simulink model "trapezgeschw_mit_statemachine"  (R2023b)
settings: Solver=ode5  StartTime=0.0  StopTime=10.0  FixedStep=1e-3  RelTol=1e-3
undefined symbols (not defined in the file or in its folder): DiscIntNeverNeededParam
settings Model: Creator=pucher  LastModifiedBy=Flo
settings SolverCC: AlgebraicLoopSolver=TrustRegion
settings DebuggingCC: UnconnectedInputMsg=warning  UnconnectedOutputMsg=warning  UnconnectedLineMsg=warning  ArithmeticOperatorsInVariantConditions=warning
settings ModelReferenceCC: EnableRefExpFcnMdlSchedulingChecks=on
settings SFSimCC: CustomCodeUndefinedFunction=UseInterfaceOnly

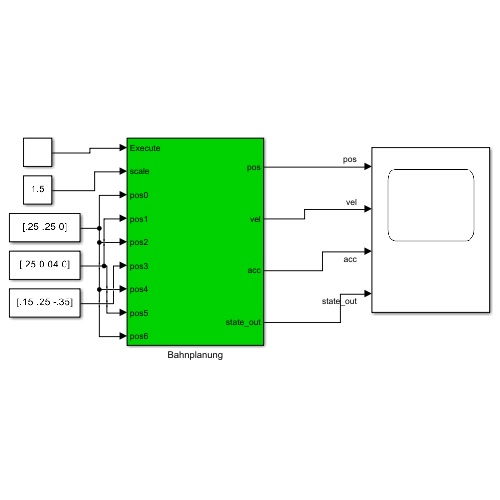
[thumbnail: Simulink's stored preview of the top-level diagram]
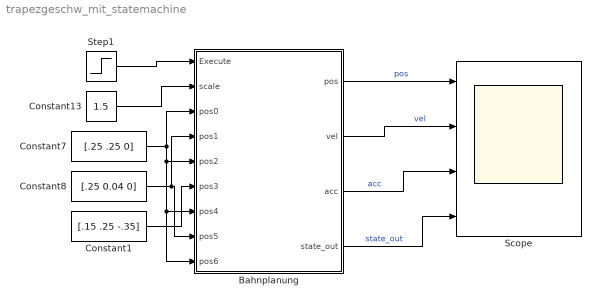
== system trapezgeschw_mit_statemachine ==
  Bahnplanung : Subsystem
  Constant1 : Constant  Value=[.15 .25 -.35]
  Constant13 : Constant  Value=1.5
  Constant7 : Constant  Value=[.25 .25 0]
  Constant8 : Constant  Value=[.25 0.04 0]
  Scope : Scope  NumInputPorts=4
  Step1 : Step
  wires:
  Constant7/1 -> Bahnplanung/9(pos6), Bahnplanung/7(pos4), Bahnplanung/5(pos2), Bahnplanung/3(pos0)
  Step1/1 -> Bahnplanung/1(Execute)
  Constant8/1 -> Bahnplanung/8(pos5), Bahnplanung/4(pos1)
  Bahnplanung/1(pos) -> Scope/1  "pos"
  Bahnplanung/2(vel) -> Scope/2  "vel"
  Bahnplanung/3(acc) -> Scope/3  "acc"
  Bahnplanung/4(state_out) -> Scope/4  "state_out"
  Constant13/1 -> Bahnplanung/2(scale)
  Constant1/1 -> Bahnplanung/6(pos3)

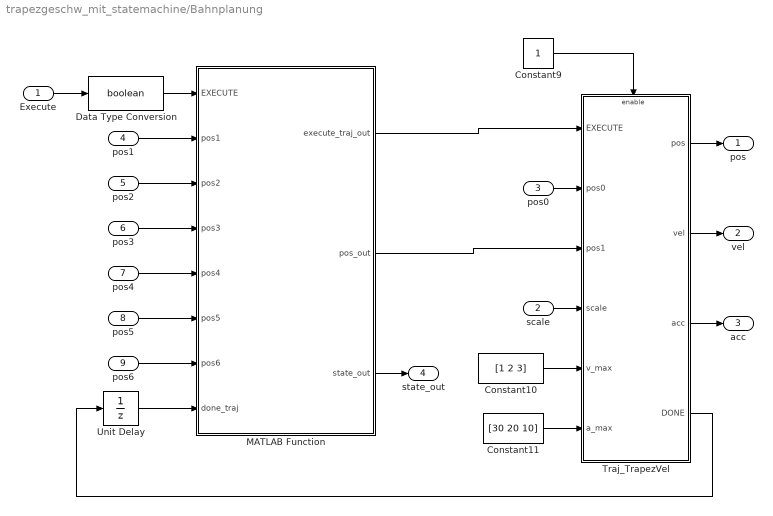
== system trapezgeschw_mit_statemachine/Bahnplanung ==
  Execute : Inport
  scale : Inport  Port=2
  pos0 : Inport  Port=3
  pos1 : Inport  Port=4
  pos2 : Inport  Port=5
  pos3 : Inport  Port=6
  pos4 : Inport  Port=7
  pos5 : Inport  Port=8
  pos6 : Inport  Port=9
  Constant10 : Constant  Value=[1 2 3]
  Constant11 : Constant  Value=[30 20 10]
  Constant9 : Constant
  Data Type Conversion : DataTypeConversion  OutDataTypeStr=boolean  SaturateOnIntegerOverflow=off  RndMeth=Floor
  MATLAB Function : MATLAB Function  TreatAsAtomicUnit=on
  Traj_TrapezVel : Subsystem
  Unit Delay : UnitDelay  SampleTime=-1  HasFrameUpgradeWarning=on
  pos : Outport
  vel : Outport  Port=2
  acc : Outport  Port=3
  state_out : Outport  Port=4
  wires:
  MATLAB Function/1(execute_traj_out) -> Traj_TrapezVel/1(EXECUTE)
  Constant10/1 -> Traj_TrapezVel/5(v_max)
  Unit Delay/1 -> MATLAB Function/8(done_traj)
  Constant9/1 -> Traj_TrapezVel/Enable
  scale/1 -> Traj_TrapezVel/4(scale)
  Traj_TrapezVel/4(DONE) -> Unit Delay/1
  Data Type Conversion/1 -> MATLAB Function/1(EXECUTE)
  Constant11/1 -> Traj_TrapezVel/6(a_max)
  Traj_TrapezVel/1(pos) -> pos/1
  Traj_TrapezVel/2(vel) -> vel/1
  MATLAB Function/2(pos_out) -> Traj_TrapezVel/3(pos1)
  MATLAB Function/3(state_out) -> state_out/1
  pos2/1 -> MATLAB Function/3(pos2)
  Execute/1 -> Data Type Conversion/1
  Traj_TrapezVel/3(acc) -> acc/1
  pos1/1 -> MATLAB Function/2(pos1)
  pos0/1 -> Traj_TrapezVel/2(pos0)
  pos4/1 -> MATLAB Function/5(pos4)
  pos5/1 -> MATLAB Function/6(pos5)
  pos3/1 -> MATLAB Function/4(pos3)
  pos6/1 -> MATLAB Function/7(pos6)

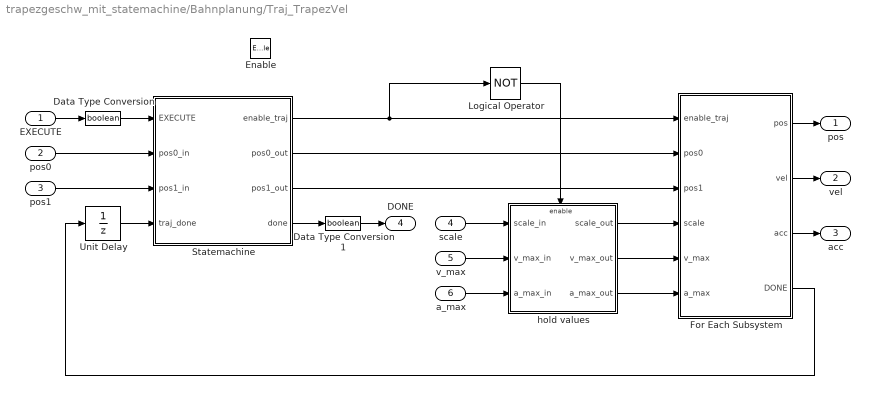
== system trapezgeschw_mit_statemachine/Bahnplanung/Traj_TrapezVel ==
  EXECUTE : Inport
  pos0 : Inport  Port=2
  pos1 : Inport  Port=3
  scale : Inport  Port=4
  v_max : Inport  Port=5
  a_max : Inport  Port=6
  Enable : EnablePort  StatesWhenEnabling=reset
  Data Type Conversion : DataTypeConversion  OutDataTypeStr=boolean  SaturateOnIntegerOverflow=off  RndMeth=Floor
  Data Type Conversion1 : DataTypeConversion  OutDataTypeStr=boolean  SaturateOnIntegerOverflow=off  RndMeth=Floor
  For Each Subsystem : Subsystem  TreatAsAtomicUnit=on
  Logical Operator : Logic  Operator=NOT  AllPortsSameDT=off  OutDataTypeStr=boolean
  Statemachine : MATLAB Function  TreatAsAtomicUnit=on
  Unit Delay : UnitDelay  SampleTime=-1  HasFrameUpgradeWarning=on
  hold values : Subsystem  TreatAsAtomicUnit=on
  pos : Outport
  vel : Outport  Port=2
  acc : Outport  Port=3
  DONE : Outport  Port=4  PortDimensions=1
  wires:
  For Each Subsystem/1(pos) -> pos/1
  For Each Subsystem/2(vel) -> vel/1
  For Each Subsystem/3(acc) -> acc/1
  Statemachine/3(pos1_out) -> For Each Subsystem/3(pos1)
  Unit Delay/1 -> Statemachine/4(traj_done)
  EXECUTE/1 -> Data Type Conversion/1
  pos0/1 -> Statemachine/2(pos0_in)
  For Each Subsystem/4(DONE) -> Unit Delay/1
  pos1/1 -> Statemachine/3(pos1_in)
  Data Type Conversion/1 -> Statemachine/1(EXECUTE)
  Statemachine/2(pos0_out) -> For Each Subsystem/2(pos0)
  Statemachine/4(done) -> Data Type Conversion1/1
  Data Type Conversion1/1 -> DONE/1
  scale/1 -> hold values/1(scale_in)
  hold values/1(scale_out) -> For Each Subsystem/4(scale)
  v_max/1 -> hold values/2(v_max_in)
  hold values/2(v_max_out) -> For Each Subsystem/5(v_max)
  a_max/1 -> hold values/3(a_max_in)
  hold values/3(a_max_out) -> For Each Subsystem/6(a_max)
  Logical Operator/1 -> hold values/Enable
  Statemachine/1(enable_traj) -> Logical Operator/1, For Each Subsystem/1(enable_traj)

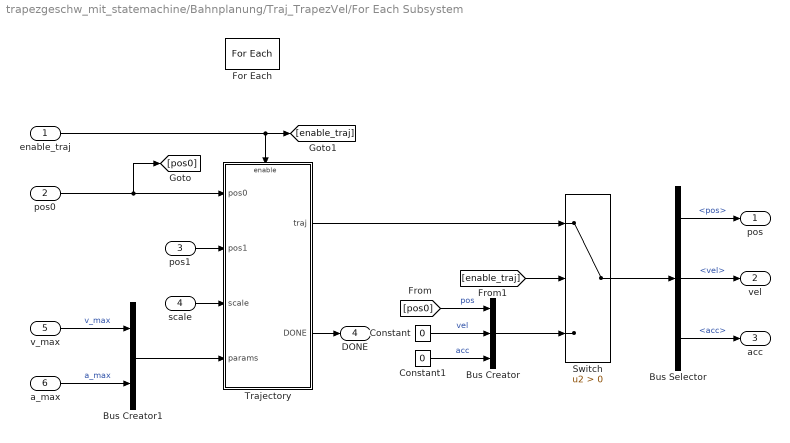
== system trapezgeschw_mit_statemachine/Bahnplanung/Traj_TrapezVel/For Each Subsystem ==
  enable_traj : Inport
  pos0 : Inport  Port=2  Partition=on  PartitionDimension=1  PartitionWidth=1  PartitionOffset=0
  pos1 : Inport  Port=3  Partition=on  PartitionDimension=1  PartitionWidth=1  PartitionOffset=0
  scale : Inport  Port=4
  v_max : Inport  Port=5  Partition=on  PartitionDimension=1  PartitionWidth=1  PartitionOffset=0
  a_max : Inport  Port=6  Partition=on  PartitionDimension=1  PartitionWidth=1  PartitionOffset=0
  Bus Creator : BusCreator  Inputs=3
  Bus Creator1 : BusCreator  Inputs=2
  Bus Selector : BusSelector  OutputSignals=pos,vel,acc
  Constant : Constant  Value=0
  Constant1 : Constant  Value=0
  For Each : ForEach  DisableCoverage=on
  Switch : Switch  Criteria=u2 > Threshold  SaturateOnIntegerOverflow=off  InputSameDT=off
  Trajectory : Subsystem
  pos : Outport  ConcatenationDimension=1
  vel : Outport  Port=2  ConcatenationDimension=1
  acc : Outport  Port=3  ConcatenationDimension=1
  DONE : Outport  Port=4  ConcatenationDimension=1  VectorParamsAs1DForOutWhenUnconnected=off
  wires:
  Constant1/1 -> Bus Creator/3  "acc"
  Constant/1 -> Bus Creator/2  "vel"
  pos1/1 -> Trajectory/2(pos1)
  Bus Creator1/1 -> Trajectory/4(params)
  Trajectory/2(DONE) -> DONE/1
  [enable_traj] -> Switch/2
  Switch/1 -> Bus Selector/1
  Bus Creator/1 -> Switch/3
  pos0/1 -> Trajectory/1(pos0), [pos0]
  Bus Selector/1 -> pos/1  "<pos>"
  v_max/1 -> Bus Creator1/1  "v_max"
  Trajectory/1(traj) -> Switch/1
  scale/1 -> Trajectory/3(scale)
  enable_traj/1 -> [enable_traj], Trajectory/Enable
  Bus Selector/2 -> vel/1  "<vel>"
  Bus Selector/3 -> acc/1  "<acc>"
  a_max/1 -> Bus Creator1/2  "a_max"
  [pos0] -> Bus Creator/1  "pos"

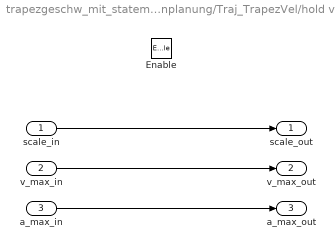
== system trapezgeschw_mit_statemachine/Bahnplanung/Traj_TrapezVel/hold values ==
  scale_in : Inport
  v_max_in : Inport  Port=2
  a_max_in : Inport  Port=3
  Enable : EnablePort
  scale_out : Outport
  v_max_out : Outport  Port=2
  a_max_out : Outport  Port=3
  wires:
  scale_in/1 -> scale_out/1
  v_max_in/1 -> v_max_out/1
  a_max_in/1 -> a_max_out/1

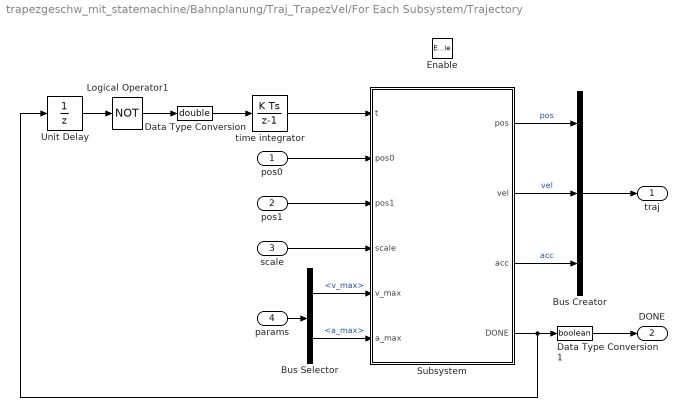
== system trapezgeschw_mit_statemachine/Bahnplanung/Traj_TrapezVel/For Each Subsystem/Trajectory ==
  pos0 : Inport  PortDimensions=1
  pos1 : Inport  Port=2  PortDimensions=1
  scale : Inport  Port=3  PortDimensions=1
  params : Inport  Port=4
  Enable : EnablePort  StatesWhenEnabling=reset
  Bus Creator : BusCreator  Inputs=3
  Bus Selector : BusSelector  OutputSignals=v_max,a_max
  Data Type Conversion : DataTypeConversion  OutDataTypeStr=double  SaturateOnIntegerOverflow=off  RndMeth=Floor
  Data Type Conversion1 : DataTypeConversion  OutDataTypeStr=boolean  SaturateOnIntegerOverflow=off  RndMeth=Floor
  Logical Operator1 : Logic  Operator=NOT  AllPortsSameDT=off  OutDataTypeStr=boolean
  Subsystem : Subsystem
  Unit Delay : UnitDelay  SampleTime=-1  HasFrameUpgradeWarning=on
  time integrator : DiscreteIntegrator  SampleTime=-1  ICPrevOutput=DiscIntNeverNeededParam  ICPrevScaledInput=DiscIntNeverNeededParam
  traj : Outport  VectorParamsAs1DForOutWhenUnconnected=off
  DONE : Outport  Port=2  PortDimensions=1  VectorParamsAs1DForOutWhenUnconnected=off
  wires:
  Data Type Conversion1/1 -> DONE/1
  params/1 -> Bus Selector/1
  Bus Creator/1 -> traj/1
  Logical Operator1/1 -> Data Type Conversion/1
  Unit Delay/1 -> Logical Operator1/1
  Data Type Conversion/1 -> time integrator/1
  Subsystem/4(DONE) -> Unit Delay/1, Data Type Conversion1/1
  time integrator/1 -> Subsystem/1(t)
  pos0/1 -> Subsystem/2(pos0)
  pos1/1 -> Subsystem/3(pos1)
  scale/1 -> Subsystem/4(scale)
  Bus Selector/1 -> Subsystem/5(v_max)  "<v_max>"
  Bus Selector/2 -> Subsystem/6(a_max)  "<a_max>"
  Subsystem/1(pos) -> Bus Creator/1  "pos"
  Subsystem/2(vel) -> Bus Creator/2  "vel"
  Subsystem/3(acc) -> Bus Creator/3  "acc"

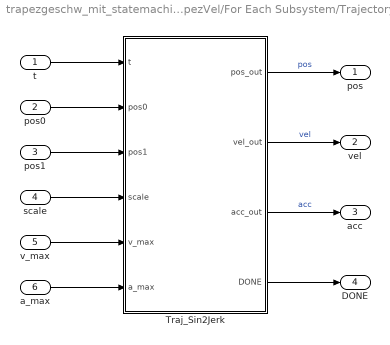
== system trapezgeschw_mit_statemachine/Bahnplanung/Traj_TrapezVel/For Each Subsystem/Trajectory/Subsystem ==
  t : Inport
  pos0 : Inport  Port=2
  pos1 : Inport  Port=3
  scale : Inport  Port=4
  v_max : Inport  Port=5
  a_max : Inport  Port=6
  Traj_Sin2Jerk : MATLAB Function  TreatAsAtomicUnit=on
  pos : Outport
  vel : Outport  Port=2
  acc : Outport  Port=3
  DONE : Outport  Port=4
  wires:
  pos0/1 -> Traj_Sin2Jerk/2(pos0)
  Traj_Sin2Jerk/1(pos_out) -> pos/1  "pos"
  a_max/1 -> Traj_Sin2Jerk/6(a_max)
  v_max/1 -> Traj_Sin2Jerk/5(v_max)
  Traj_Sin2Jerk/3(acc_out) -> acc/1  "acc"
  Traj_Sin2Jerk/4(DONE) -> DONE/1
  pos1/1 -> Traj_Sin2Jerk/3(pos1)
  t/1 -> Traj_Sin2Jerk/1(t)
  Traj_Sin2Jerk/2(vel_out) -> vel/1  "vel"
  scale/1 -> Traj_Sin2Jerk/4(scale)

== matlab function trapezgeschw_mit_statemachine/Bahnplanung/MATLAB Function ==
  data: execute_traj_out output; pos_out output; EXECUTE input; state_out output; pos1 input; pos2 input; pos3 input; pos4 input; pos5 input; pos6 input; done_traj input
function [execute_traj_out, pos_out, state_out] = Statemachine(EXECUTE, pos1, pos2, pos3, pos4, pos5, pos6, done_traj)

    persistent state prev_execute dest_pos execute_traj;

    % initializations
    STATE_INIT = 0;
    STATE_TRAJ1 = 10;
    STATE_TRAJ2 = 20;
    STATE_TRAJ3 = 30;
    STATE_TRAJ4 = 40;
    STATE_TRAJ5 = 50;
    STATE_TRAJ6 = 60;
    STATE_DONE = 70;

    if(isempty(state))
        state = STATE_INIT;
        prev_execute = false;
        execute_traj = false;
        dest_pos = pos1;
    end

    % state machine
    switch(state)
        case STATE_INIT
            execute_traj = false;
            if EXECUTE && ~prev_execute
                state = STATE_TRAJ1;
            end
        case STATE_TRAJ1
            execute_traj = true;
            dest_pos = pos1;
            if done_traj
                execute_traj = false;
                state = STATE_TRAJ2;
            end
        case STATE_TRAJ2
            execute_traj = true;
            dest_pos = pos2;
            if done_traj
                execute_traj = false;
                state = STATE_TRAJ3;
            end
        case STATE_TRAJ3
            execute_traj = true;
            dest_pos = pos3;
            if done_traj
                execute_traj = false;
                state = STATE_TRAJ4;
            end
        case STATE_TRAJ4
            execute_traj = true;
            dest_pos = pos4;
            if done_traj
                execute_traj = false;
                state = STATE_TRAJ5;
            end
        case STATE_TRAJ5
            execute_traj = true;
            dest_pos = pos5;
            if done_traj
                execute_traj = false;
                state = STATE_TRAJ6;
            end
        case STATE_TRAJ6
            execute_traj = true;
            dest_pos = pos6;
            if done_traj
                execute_traj = false;
                state = STATE_DONE;
            end
        case STATE_DONE
            execute_traj = false;
            % FINISHED
    end
    prev_execute = EXECUTE;
    state_out = state;
    execute_traj_out = execute_traj;
    pos_out = dest_pos;
end

== matlab function trapezgeschw_mit_statemachine/Bahnplanung/Traj_TrapezVel/For Each Subsystem/Trajectory/Subsystem/Traj_Sin2Jerk ==
  data: t input; pos_out output; pos0 input; pos1 input; scale input; v_max input; a_max input; vel_out output; acc_out output; DONE output
function [ pos_out, vel_out, acc_out, DONE] = emf_Traj_TrapezVel(t, pos0, pos1, scale, v_max, a_max)

	t = scale * t;
	
	[pos, vel, acc, t_end ] = Traj_TrapezVel(t, pos0, pos1, v_max, a_max); 

	pos_out  = pos;
	vel_out  = vel  * scale;
	acc_out  = acc  * scale * scale; % scale^2
    
	if t >= t_end
		DONE = true;
	else
		DONE = false;
	end

end

== matlab function trapezgeschw_mit_statemachine/Bahnplanung/Traj_TrapezVel/Statemachine ==
  data: EXECUTE input; enable_traj output; pos0_in input; pos1_in input; traj_done input; pos0_out output; pos1_out output; done output
function [enable_traj, pos0_out, pos1_out, done] = Statemachine(EXECUTE, pos0_in, pos1_in, traj_done)
    
	persistent state pos0 pos1 prev_execute

	STATE_INIT = 0;
	STATE_MOVE = 10;
	STATE_DONE = 20;

	if isempty(state)
		state = STATE_INIT;
		pos0 = pos0_in;
		pos1 = pos0_in;
		prev_execute = false;
	end
    
    enable_traj = false;
	done = false;

	switch state
		case STATE_INIT
			if EXECUTE && ~prev_execute
                pos1 = pos1_in;
                state = STATE_MOVE;
                enable_traj = true;
			end

		case STATE_MOVE
			enable_traj = true;
			if all(traj_done)
				state = STATE_DONE;
				done = true;
			end

		case STATE_DONE
			enable_traj = true;
			done = true;
            if ~EXECUTE
				state = STATE_INIT;
				pos0 = pos1;
				enable_traj = false;
				done = false;
            end
	end
	prev_execute = EXECUTE;
	pos0_out = pos0;
	pos1_out = pos1;

end
